simulink model "uavclosed"  (R2022b)
settings: Solver=VariableStepAuto  StartTime=0.0  StopTime=30  RelTol=1e-3
libraries: slpidlib x2, simulink x1
settings Model: Creator=Zzera  LastModifiedBy=Zzera

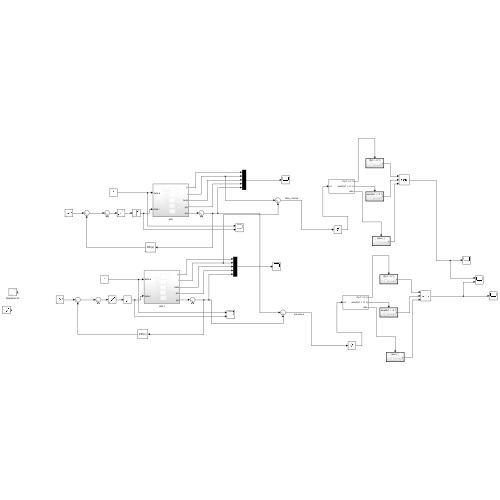
[thumbnail: Simulink's stored preview of the top-level diagram]
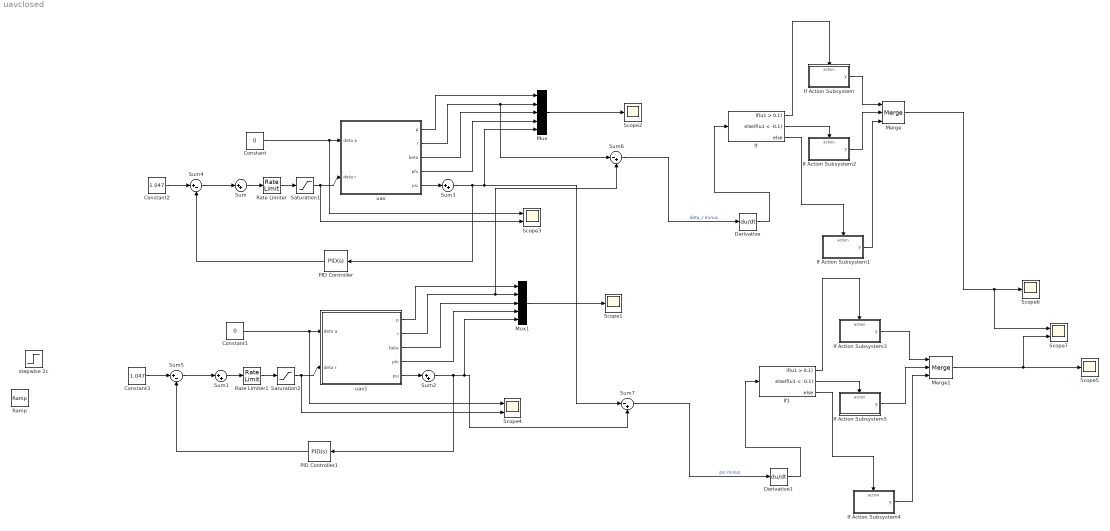
== system uavclosed ==
  Constant : Constant  Value=0
  Constant1 : Constant  Value=0
  Constant2 : Constant  Value=1.047
  Constant3 : Constant  Value=1.047
  Derivative : Derivative
  Derivative1 : Derivative
  If : If  IfExpression=u1 > 0.1  ElseIfExpressions=u1 < -0.1  ZeroCross=off
  If Action Subsystem : Subsystem  TreatAsAtomicUnit=on
  If Action Subsystem1 : Subsystem  TreatAsAtomicUnit=on
  If Action Subsystem2 : Subsystem  TreatAsAtomicUnit=on
  If Action Subsystem3 : Subsystem  TreatAsAtomicUnit=on
  If Action Subsystem4 : Subsystem  TreatAsAtomicUnit=on
  If Action Subsystem5 : Subsystem  TreatAsAtomicUnit=on
  If1 : If  IfExpression=u1 > 0.1  ElseIfExpressions=u1 < -0.1  ZeroCross=off
  Merge : Merge  Inputs=3
  Merge1 : Merge  Inputs=3
  Mux : Mux  Inputs=5
  Mux1 : Mux  Inputs=5
  PID Controller : slpidlib/PID Controller  Controller=PID  Form=Parallel  TimeDomain=Continuous-time  UseExternalTs=off  SampleTime=-1  IntegratorMethod=Forward Euler  FilterMethod=Forward Euler  ControllerParametersSource=internal  P=1  I=0  UseKiTs=off  D=0  N=100  UseFilter=on  TunerSelectOption=Transfer Function Based (PID Tuner App)  InitialConditionSource=internal  InitialConditionForIntegrator=0  InitialConditionForFilter=0  DifferentiatorICPrevScaledInput=0  ExternalReset=none  TrackingMode=off  Kt=1  LimitOutput=off  SatLimitsSource=internal  UpperSaturationLimit=inf  LowerSaturationLimit=-inf  LinearizeAsGain=on  AntiWindupMode=none  Kb=1  LimitIntegrator=off  UpperIntegratorSaturationLimit=inf  LowerIntegratorSaturationLimit=-inf  POutMin=[]  POutMax=[]  IOutMin=[]  IOutMax=[]  DOutMin=[]  DOutMax=[]  NOutMin=[]  NOutMax=[]  SumOutMin=[]  SumOutMax=[]  SaturationOutMin=[]  SaturationOutMax=[]  PParamMin=[]  PParamMax=[]  IParamMin=[]  IParamMax=[]  DParamMin=[]  DParamMax=[]  NParamMin=[]  NParamMax=[]  KbParamMin=[]  KbParamMax=[]  KtParamMin=[]  KtParamMax=[]  KbOutMin=[]  KbOutMax=[]  KtOutMin=[]  KtOutMax=[]  IntegratorOutMin=[]  IntegratorOutMax=[]  FilterOutMin=[]  FilterOutMax=[]  SumI1OutMin=[]  SumI1OutMax=[]  SumI2OutMin=[]  SumI2OutMax=[]  SumI3OutMin=[]  SumI3OutMax=[]  SumI4OutMin=[]  SumI4OutMax=[]  SumDOutMin=[]  SumDOutMax=[]  DifferentiatorOutMin=[]  DifferentiatorOutMax=[]  FilterDiffOutCoefMin=[]  FilterDiffOutCoefMax=[]  ReciprocalOutMin=[]  ReciprocalOutMax=[]  SumDenOutMin=[]  SumDenOutMax=[]  SumNumOutMin=[]  SumNumOutMax=[]  DivideOutMin=[]  DivideOutMax=[]  UdiffTsProdOutMin=[]  UdiffTsProdOutMax=[]  NTsProdOutMin=[]  NTsProdOutMax=[]  UintegralTsProdOutMin=[]  UintegralTsProdOutMax=[]  UngainTsProdOutMin=[]  UngainTsProdOutMax=[]  ClampingZeroOutDataTypeStr=Inherit: Inherit via back propagation  ClampingZeroOutMin=[]  ClampingZeroOutMax=[]  FilterDenConstantOutDataTypeStr=Inherit: Inherit via back propagation  FilterDenConstantOutMin=[]  FilterDenConstantOutMax=[]  PCopyOutDataTypeStr=Inherit: Inherit via back propagation  PCopyOutMin=[]  PCopyOutMax=[]  NCopyOutDataTypeStr=Inherit: Inherit via back propagation  NCopyOutMin=[]  NCopyOutMax=[]  IntegratorContinuousStateAttributes=''  IntegratorStateMustResolveToSignalObject=off  IntegratorRTWStateStorageClass=Auto  FilterContinuousStateAttributes=''  FilterStateMustResolveToSignalObject=off  FilterRTWStateStorageClass=Auto  ParallelPVariant=InternalParameters  IdealPVariant=Disabled  IVariant=InternalParameters  DVariant=InternalParameters  IntegratorVariant=Continuous  SatVariant=Disabled  AWVariant=Passthrough  PCopyVariant=Disabled  TRVariant=Disabled  FdbkBlocksVariant=Forward  IdealPFdbkVariant=Disabled  SatFdbkVariant=Disabled  DerivativeFilterVariant=ContFilter  NVariant=InternalParameters  NCopyVariant=Disabled  FilterICVariant=InternalICsFilter  IntegratorICVariant=InternalICs  ExternalResetVariant=Disabled  TRSumVariant=Passthrough  SumFdbkVariant=Disabled  SumVariant=Sum_PID  TsampFilterVariant=InternalTs  TsampNgainVariant=Passthrough  TsampIntegralVariant=Passthrough  ExternalSaturationOutDataTypeStr=Inherit: Same as second input
  PID Controller1 : slpidlib/PID Controller  Controller=PID  Form=Parallel  TimeDomain=Continuous-time  UseExternalTs=off  SampleTime=-1  IntegratorMethod=Forward Euler  FilterMethod=Forward Euler  ControllerParametersSource=internal  P=1  I=0  UseKiTs=off  D=0  N=100  UseFilter=on  TunerSelectOption=Transfer Function Based (PID Tuner App)  InitialConditionSource=internal  InitialConditionForIntegrator=0  InitialConditionForFilter=0  DifferentiatorICPrevScaledInput=0  ExternalReset=none  TrackingMode=off  Kt=1  LimitOutput=off  SatLimitsSource=internal  UpperSaturationLimit=inf  LowerSaturationLimit=-inf  LinearizeAsGain=on  AntiWindupMode=none  Kb=1  LimitIntegrator=off  UpperIntegratorSaturationLimit=inf  LowerIntegratorSaturationLimit=-inf  POutMin=[]  POutMax=[]  IOutMin=[]  IOutMax=[]  DOutMin=[]  DOutMax=[]  NOutMin=[]  NOutMax=[]  SumOutMin=[]  SumOutMax=[]  SaturationOutMin=[]  SaturationOutMax=[]  PParamMin=[]  PParamMax=[]  IParamMin=[]  IParamMax=[]  DParamMin=[]  DParamMax=[]  NParamMin=[]  NParamMax=[]  KbParamMin=[]  KbParamMax=[]  KtParamMin=[]  KtParamMax=[]  KbOutMin=[]  KbOutMax=[]  KtOutMin=[]  KtOutMax=[]  IntegratorOutMin=[]  IntegratorOutMax=[]  FilterOutMin=[]  FilterOutMax=[]  SumI1OutMin=[]  SumI1OutMax=[]  SumI2OutMin=[]  SumI2OutMax=[]  SumI3OutMin=[]  SumI3OutMax=[]  SumI4OutMin=[]  SumI4OutMax=[]  SumDOutMin=[]  SumDOutMax=[]  DifferentiatorOutMin=[]  DifferentiatorOutMax=[]  FilterDiffOutCoefMin=[]  FilterDiffOutCoefMax=[]  ReciprocalOutMin=[]  ReciprocalOutMax=[]  SumDenOutMin=[]  SumDenOutMax=[]  SumNumOutMin=[]  SumNumOutMax=[]  DivideOutMin=[]  DivideOutMax=[]  UdiffTsProdOutMin=[]  UdiffTsProdOutMax=[]  NTsProdOutMin=[]  NTsProdOutMax=[]  UintegralTsProdOutMin=[]  UintegralTsProdOutMax=[]  UngainTsProdOutMin=[]  UngainTsProdOutMax=[]  ClampingZeroOutDataTypeStr=Inherit: Inherit via back propagation  ClampingZeroOutMin=[]  ClampingZeroOutMax=[]  FilterDenConstantOutDataTypeStr=Inherit: Inherit via back propagation  FilterDenConstantOutMin=[]  FilterDenConstantOutMax=[]  PCopyOutDataTypeStr=Inherit: Inherit via back propagation  PCopyOutMin=[]  PCopyOutMax=[]  NCopyOutDataTypeStr=Inherit: Inherit via back propagation  NCopyOutMin=[]  NCopyOutMax=[]  IntegratorContinuousStateAttributes=''  IntegratorStateMustResolveToSignalObject=off  IntegratorRTWStateStorageClass=Auto  FilterContinuousStateAttributes=''  FilterStateMustResolveToSignalObject=off  FilterRTWStateStorageClass=Auto  ParallelPVariant=InternalParameters  IdealPVariant=Disabled  IVariant=InternalParameters  DVariant=InternalParameters  IntegratorVariant=Continuous  SatVariant=Disabled  AWVariant=Passthrough  PCopyVariant=Disabled  TRVariant=Disabled  FdbkBlocksVariant=Forward  IdealPFdbkVariant=Disabled  SatFdbkVariant=Disabled  DerivativeFilterVariant=ContFilter  NVariant=InternalParameters  NCopyVariant=Disabled  FilterICVariant=InternalICsFilter  IntegratorICVariant=InternalICs  ExternalResetVariant=Disabled  TRSumVariant=Passthrough  SumFdbkVariant=Disabled  SumVariant=Sum_PID  TsampFilterVariant=InternalTs  TsampNgainVariant=Passthrough  TsampIntegralVariant=Passthrough  ExternalSaturationOutDataTypeStr=Inherit: Same as second input
  Ramp : simulink/Sources/Ramp  slope=0.4  start=10  InitialOutput=0
  Rate Limiter : RateLimiter  RisingSlewLimit=0.3491  FallingSlewLimit=-0.3491
  Rate Limiter1 : RateLimiter  RisingSlewLimit=0.3491  FallingSlewLimit=-0.3491
  Saturation1 : Saturate  UpperLimit=1.308  LowerLimit=-1.308
  Saturation2 : Saturate  UpperLimit=1.308  LowerLimit=-1.308
  Scope{1..2,5..6} (4 alike) : Scope
  Scope3 : Scope  NumInputPorts=2
  Scope4 : Scope  NumInputPorts=2
  Scope7 : Scope  NumInputPorts=2
  Sum{,1..3} (4 alike) : Sum  Inputs=|++
  Sum4 : Sum  Inputs=|+-
  Sum5 : Sum  Inputs=|+-
  Sum6 : Sum  Inputs=|-+
  Sum7 : Sum  Inputs=|-+
  stepwise 2c : Step  After=0.2  SampleTime=10
  uav : Subsystem
  uav1 : Subsystem
  wires:
  Constant/1 -> Scope3/1, uav/1(deta a)
  uav/2(r) -> Sum6/1, Mux/2
  uav/5(psi) -> Sum3/1
  uav/1(p) -> Mux/1
  uav/3(beta) -> Mux/3
  uav/4(phi) -> Mux/4
  Mux/1 -> Scope2/1
  Sum3/1 -> PID Controller/1, Sum7/1, Mux/5
  Saturation1/1 -> Scope3/2, uav/2(deta r)
  Sum/1 -> Rate Limiter/1
  Rate Limiter/1 -> Saturation1/1
  Constant2/1 -> Sum4/1
  Sum4/1 -> Sum/1
  PID Controller/1 -> Sum4/2
  Sum1/1 -> Rate Limiter1/1
  uav1/1(p) -> Mux1/1
  Mux1/1 -> Scope1/1
  PID Controller1/1 -> Sum5/2
  Constant3/1 -> Sum5/1
  uav1/5(psi) -> Sum2/1
  Sum2/1 -> PID Controller1/1, Sum7/2, Mux1/5
  Constant1/1 -> Scope4/1, uav1/1(deta a)
  Rate Limiter1/1 -> Saturation2/1
  uav1/2(r) -> Sum6/2, Mux1/2
  uav1/4(phi) -> Mux1/4
  Saturation2/1 -> Scope4/2, uav1/2(deta r)
  uav1/3(beta) -> Mux1/3
  Sum5/1 -> Sum1/1
  If Action Subsystem2/1(y) -> Merge/2
  If1/3 -> If Action Subsystem4/Action
  If Action Subsystem1/1(y) -> Merge/3
  If1/2 -> If Action Subsystem5/Action
  If Action Subsystem4/1(y) -> Merge1/3
  Derivative/1 -> If/1
  If/3 -> If Action Subsystem1/Action
  If/1 -> If Action Subsystem/Action
  Sum6/1 -> Derivative/1  "deta_r minus"
  Merge/1 -> Scope7/1, Scope6/1
  Sum7/1 -> Derivative1/1  "psi minus"
  Derivative1/1 -> If1/1
  If Action Subsystem5/1(y) -> Merge1/2
  If/2 -> If Action Subsystem2/Action
  Merge1/1 -> Scope7/2, Scope5/1
  If1/1 -> If Action Subsystem3/Action
  If Action Subsystem3/1(y) -> Merge1/1
  If Action Subsystem/1(y) -> Merge/1

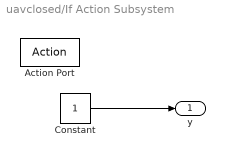
== system uavclosed/If Action Subsystem ==
  Action Port : ActionPort  ActionPortLabel=if(u1 > 0.1)
  Constant : Constant
  y : Outport
  wires:
  Constant/1 -> y/1

== system uavclosed/If Action Subsystem1 ==
  Action Port : ActionPort  ActionPortLabel=else
  Constant : Constant  Value=0
  y : Outport
  wires:
  Constant/1 -> y/1

== system uavclosed/If Action Subsystem2 ==
  Action Port : ActionPort  ActionPortLabel=elseif(u1 < -0.1)
  Constant : Constant
  y : Outport
  wires:
  Constant/1 -> y/1

== system uavclosed/If Action Subsystem3 ==
  Action Port : ActionPort  ActionPortLabel=if(u1 > 0.1)
  Constant : Constant
  y : Outport
  wires:
  Constant/1 -> y/1

== system uavclosed/If Action Subsystem4 ==
  Action Port : ActionPort  ActionPortLabel=else
  Constant : Constant  Value=0
  y : Outport
  wires:
  Constant/1 -> y/1

== system uavclosed/If Action Subsystem5 ==
  Action Port : ActionPort  ActionPortLabel=elseif(u1 < -0.1)
  Constant : Constant
  y : Outport
  wires:
  Constant/1 -> y/1

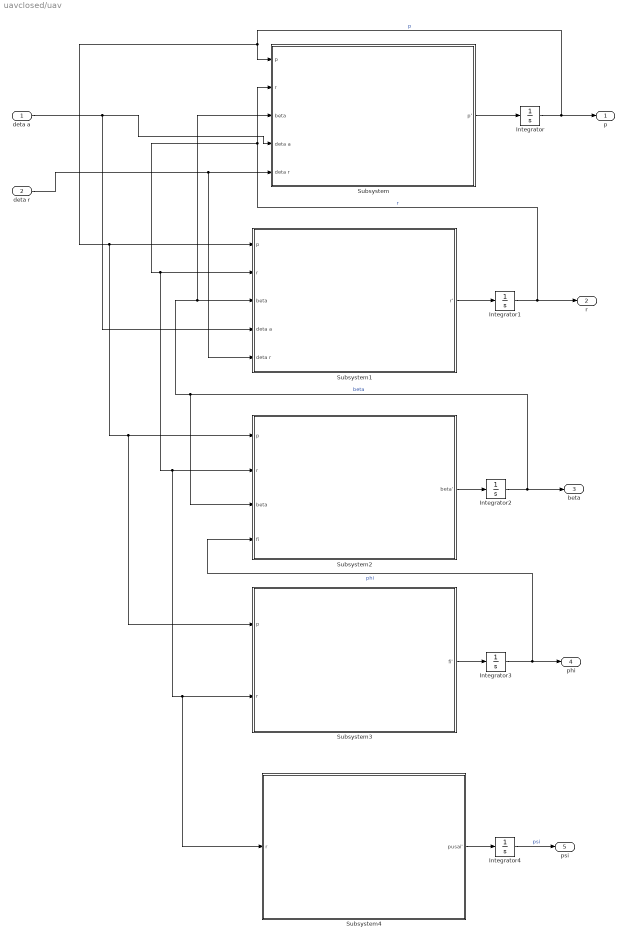
== system uavclosed/uav ==
  deta a : Inport
  deta r : Inport  Port=2
  Integrator{,1..4} (5 alike) : Integrator
  Subsystem : Subsystem
  Subsystem1 : Subsystem
  Subsystem2 : Subsystem
  Subsystem3 : Subsystem
  Subsystem4 : Subsystem
  p : Outport
  r : Outport  Port=2
  beta : Outport  Port=3
  phi : Outport  Port=4
  psi : Outport  Port=5
  wires:
  Integrator4/1 -> psi/1  "psi"
  Integrator3/1 -> phi/1, Subsystem2/4(fi)  "phi"
  Subsystem/1(p') -> Integrator/1
  Subsystem3/1(fi') -> Integrator3/1
  Integrator/1 -> p/1, Subsystem3/1(p), Subsystem2/1(p), Subsystem1/1(p), Subsystem/1(p)  "p"
  Subsystem2/1(beta') -> Integrator2/1
  Integrator1/1 -> r/1, Subsystem/2(r), Subsystem4/1(r), Subsystem3/2(r), Subsystem2/2(r), Subsystem1/2(r)  "r"
  Subsystem4/1(pusai') -> Integrator4/1
  Integrator2/1 -> beta/1, Subsystem2/3(beta), Subsystem/3(beta), Subsystem1/3(beta)  "beta"
  Subsystem1/1(r') -> Integrator1/1
  deta a/1 -> Subsystem1/4(deta a), Subsystem/4(deta a)
  deta r/1 -> Subsystem1/5(deta r), Subsystem/5(deta r)

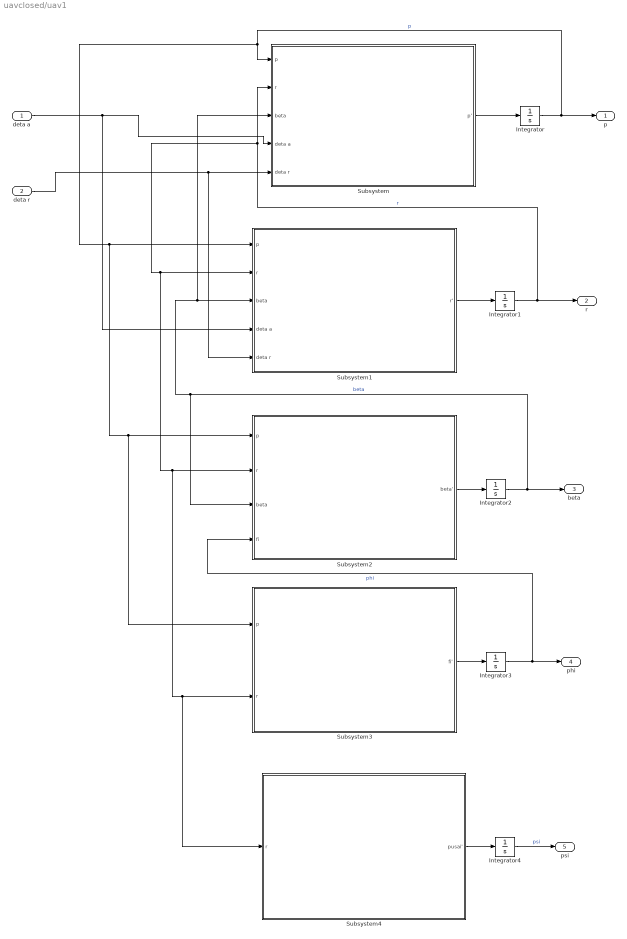
== system uavclosed/uav1 ==
  deta a : Inport
  deta r : Inport  Port=2
  Integrator{,1..4} (5 alike) : Integrator
  Subsystem : Subsystem
  Subsystem1 : Subsystem
  Subsystem2 : Subsystem
  Subsystem3 : Subsystem
  Subsystem4 : Subsystem
  p : Outport
  r : Outport  Port=2
  beta : Outport  Port=3
  phi : Outport  Port=4
  psi : Outport  Port=5
  wires:
  Integrator4/1 -> psi/1  "psi"
  Integrator3/1 -> phi/1, Subsystem2/4(fi)  "phi"
  Subsystem/1(p') -> Integrator/1
  Subsystem3/1(fi') -> Integrator3/1
  Integrator/1 -> p/1, Subsystem3/1(p), Subsystem2/1(p), Subsystem1/1(p), Subsystem/1(p)  "p"
  Subsystem2/1(beta') -> Integrator2/1
  Integrator1/1 -> r/1, Subsystem/2(r), Subsystem4/1(r), Subsystem3/2(r), Subsystem2/2(r), Subsystem1/2(r)  "r"
  Subsystem4/1(pusai') -> Integrator4/1
  Integrator2/1 -> beta/1, Subsystem2/3(beta), Subsystem/3(beta), Subsystem1/3(beta)  "beta"
  Subsystem1/1(r') -> Integrator1/1
  deta a/1 -> Subsystem1/4(deta a), Subsystem/4(deta a)
  deta r/1 -> Subsystem1/5(deta r), Subsystem/5(deta r)

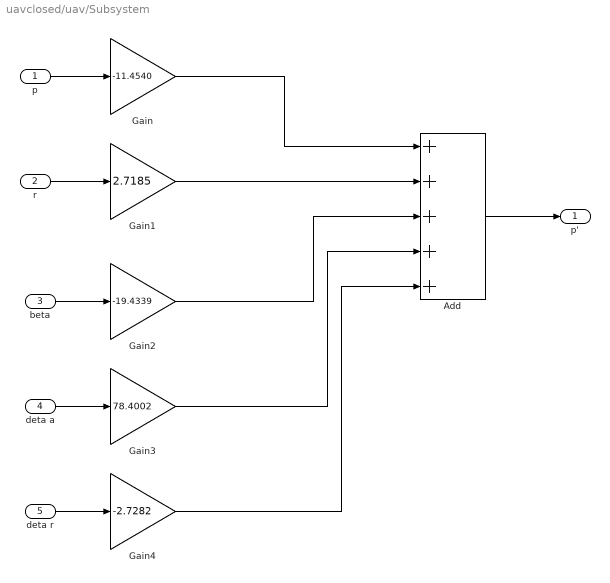
== system uavclosed/uav/Subsystem ==
  p : Inport
  r : Inport  Port=2
  beta : Inport  Port=3
  deta a : Inport  Port=4
  deta r : Inport  Port=5
  Add : Sum  Inputs=+++++
  Gain : Gain  Gain=-11.4540
  Gain1 : Gain  Gain=2.7185
  Gain2 : Gain  Gain=-19.4339
  Gain3 : Gain  Gain=78.4002
  Gain4 : Gain  Gain=-2.7282
  p' : Outport
  wires:
  Gain2/1 -> Add/3
  Gain3/1 -> Add/4
  Gain/1 -> Add/1
  Gain1/1 -> Add/2
  Gain4/1 -> Add/5
  p/1 -> Gain/1
  r/1 -> Gain1/1
  beta/1 -> Gain2/1
  deta a/1 -> Gain3/1
  deta r/1 -> Gain4/1
  Add/1 -> p'/1

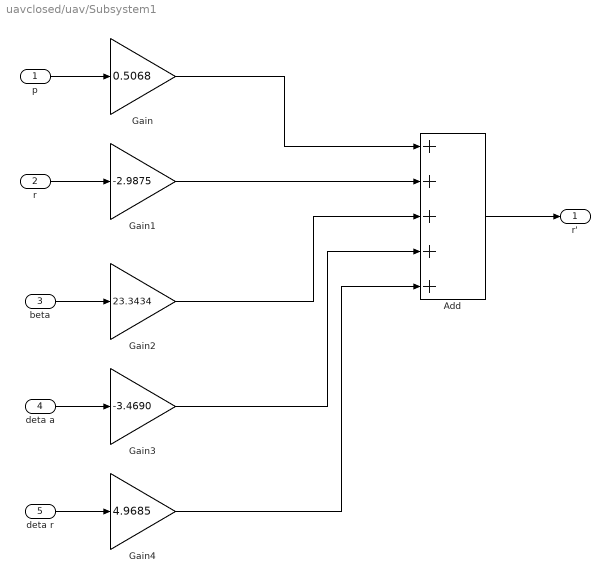
== system uavclosed/uav/Subsystem1 ==
  p : Inport
  r : Inport  Port=2
  beta : Inport  Port=3
  deta a : Inport  Port=4
  deta r : Inport  Port=5
  Add : Sum  Inputs=+++++
  Gain : Gain  Gain=0.5068
  Gain1 : Gain  Gain=-2.9875
  Gain2 : Gain  Gain=23.3434
  Gain3 : Gain  Gain=-3.4690
  Gain4 : Gain  Gain=4.9685
  r' : Outport
  wires:
  p/1 -> Gain/1
  Gain4/1 -> Add/5
  Gain1/1 -> Add/2
  Gain/1 -> Add/1
  Gain2/1 -> Add/3
  beta/1 -> Gain2/1
  Gain3/1 -> Add/4
  deta a/1 -> Gain3/1
  Add/1 -> r'/1
  deta r/1 -> Gain4/1
  r/1 -> Gain1/1

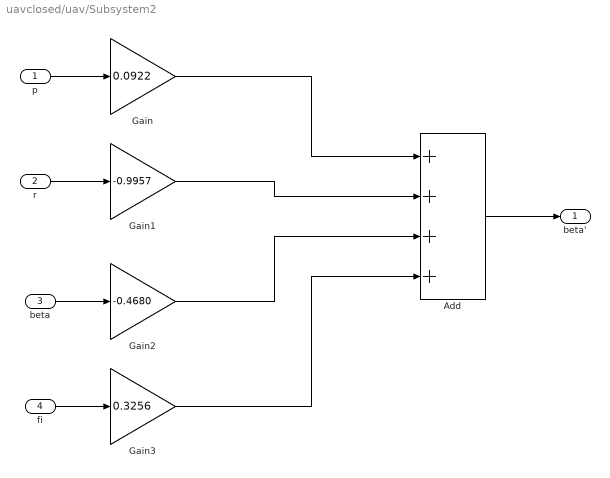
== system uavclosed/uav/Subsystem2 ==
  p : Inport
  r : Inport  Port=2
  beta : Inport  Port=3
  fi : Inport  Port=4
  Add : Sum  Inputs=++++
  Gain : Gain  Gain=0.0922
  Gain1 : Gain  Gain=-0.9957
  Gain2 : Gain  Gain=-0.4680
  Gain3 : Gain  Gain=0.3256
  beta' : Outport
  wires:
  p/1 -> Gain/1
  Gain1/1 -> Add/2
  Gain/1 -> Add/1
  Gain2/1 -> Add/3
  beta/1 -> Gain2/1
  Gain3/1 -> Add/4
  fi/1 -> Gain3/1
  Add/1 -> beta'/1
  r/1 -> Gain1/1

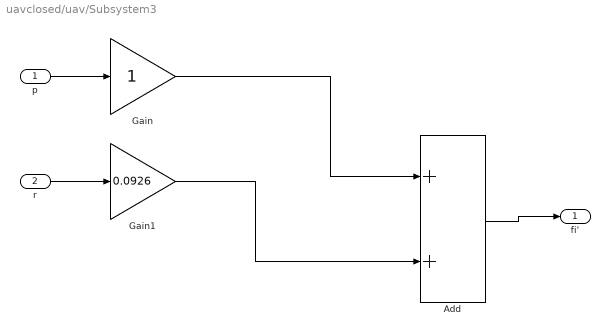
== system uavclosed/uav/Subsystem3 ==
  p : Inport
  r : Inport  Port=2
  Add : Sum
  Gain : Gain
  Gain1 : Gain  Gain=0.0926
  fi' : Outport
  wires:
  p/1 -> Gain/1
  Gain1/1 -> Add/2
  Gain/1 -> Add/1
  Add/1 -> fi'/1
  r/1 -> Gain1/1

== system uavclosed/uav/Subsystem4 ==
  r : Inport
  Gain1 : Gain
  pusai' : Outport
  wires:
  r/1 -> Gain1/1
  Gain1/1 -> pusai'/1

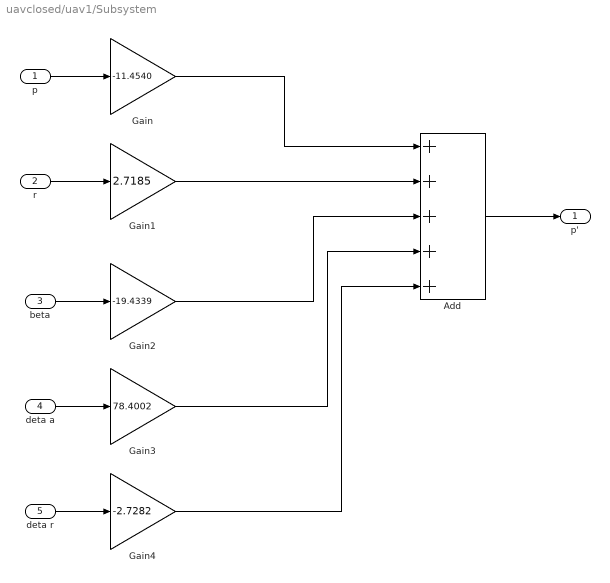
== system uavclosed/uav1/Subsystem ==
  p : Inport
  r : Inport  Port=2
  beta : Inport  Port=3
  deta a : Inport  Port=4
  deta r : Inport  Port=5
  Add : Sum  Inputs=+++++
  Gain : Gain  Gain=-11.4540
  Gain1 : Gain  Gain=2.7185
  Gain2 : Gain  Gain=-19.4339
  Gain3 : Gain  Gain=78.4002
  Gain4 : Gain  Gain=-2.7282
  p' : Outport
  wires:
  Gain2/1 -> Add/3
  Gain3/1 -> Add/4
  Gain/1 -> Add/1
  Gain1/1 -> Add/2
  Gain4/1 -> Add/5
  p/1 -> Gain/1
  r/1 -> Gain1/1
  beta/1 -> Gain2/1
  deta a/1 -> Gain3/1
  deta r/1 -> Gain4/1
  Add/1 -> p'/1

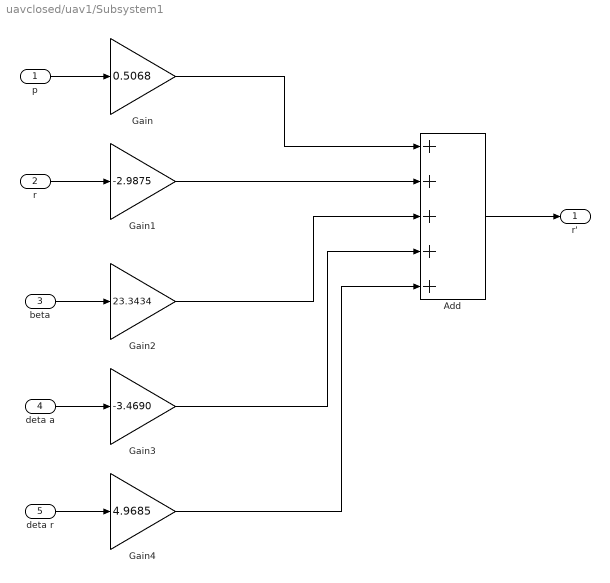
== system uavclosed/uav1/Subsystem1 ==
  p : Inport
  r : Inport  Port=2
  beta : Inport  Port=3
  deta a : Inport  Port=4
  deta r : Inport  Port=5
  Add : Sum  Inputs=+++++
  Gain : Gain  Gain=0.5068
  Gain1 : Gain  Gain=-2.9875
  Gain2 : Gain  Gain=23.3434
  Gain3 : Gain  Gain=-3.4690
  Gain4 : Gain  Gain=4.9685
  r' : Outport
  wires:
  p/1 -> Gain/1
  Gain4/1 -> Add/5
  Gain1/1 -> Add/2
  Gain/1 -> Add/1
  Gain2/1 -> Add/3
  beta/1 -> Gain2/1
  Gain3/1 -> Add/4
  deta a/1 -> Gain3/1
  Add/1 -> r'/1
  deta r/1 -> Gain4/1
  r/1 -> Gain1/1

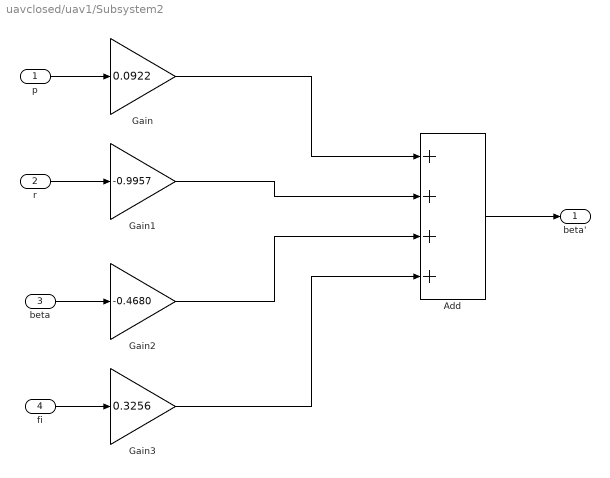
== system uavclosed/uav1/Subsystem2 ==
  p : Inport
  r : Inport  Port=2
  beta : Inport  Port=3
  fi : Inport  Port=4
  Add : Sum  Inputs=++++
  Gain : Gain  Gain=0.0922
  Gain1 : Gain  Gain=-0.9957
  Gain2 : Gain  Gain=-0.4680
  Gain3 : Gain  Gain=0.3256
  beta' : Outport
  wires:
  p/1 -> Gain/1
  Gain1/1 -> Add/2
  Gain/1 -> Add/1
  Gain2/1 -> Add/3
  beta/1 -> Gain2/1
  Gain3/1 -> Add/4
  fi/1 -> Gain3/1
  Add/1 -> beta'/1
  r/1 -> Gain1/1

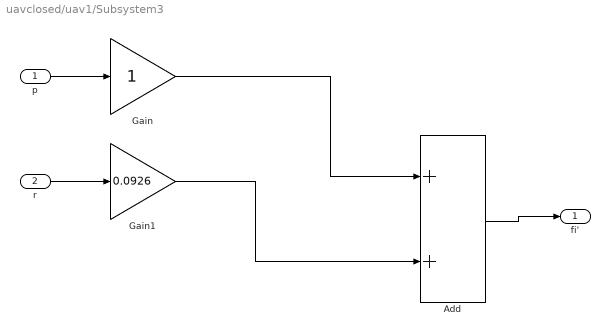
== system uavclosed/uav1/Subsystem3 ==
  p : Inport
  r : Inport  Port=2
  Add : Sum
  Gain : Gain
  Gain1 : Gain  Gain=0.0926
  fi' : Outport
  wires:
  p/1 -> Gain/1
  Gain1/1 -> Add/2
  Gain/1 -> Add/1
  Add/1 -> fi'/1
  r/1 -> Gain1/1

== system uavclosed/uav1/Subsystem4 ==
  r : Inport
  Gain1 : Gain
  pusai' : Outport
  wires:
  r/1 -> Gain1/1
  Gain1/1 -> pusai'/1
